simulink model "vehicle5a"  (R2017a)
settings: Solver=VariableStepAuto  StartTime=0.0  StopTime=2  RelTol=1e-3
libraries: elvio x6
settings Model: Creator=tstef  LastModifiedBy=tstef

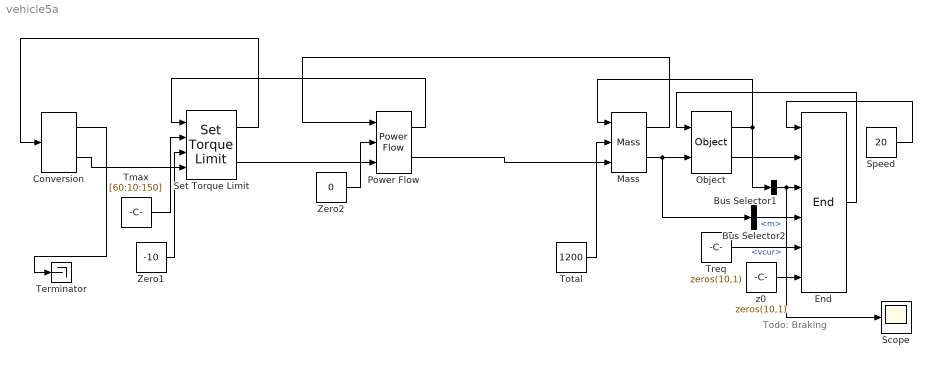
== system vehicle5a ==
  note: Todo: Braking
  Bus Selector1 : BusSelector  OutputSignals=vcur
  Bus Selector2 : BusSelector  OutputSignals=m
  Conversion : elvio/Basics/Conversion
  End : elvio/Basics/End
  Mass : elvio/Basics/Mass
  Object : elvio/Basics/Object
  Power Flow : elvio/Basics/Power Flow
  Scope : Scope
  Set Torque Limit : elvio/Basics/Set Torque Limit
  Speed : Constant  Value=20
  Terminator : Terminator
  Tmax : Constant  Value=[60:10:150]
  Total : Constant  Value=1200
  Treq : Constant  Value=zeros(10,1)
  Zero1 : Constant  Value=-10
  Zero2 : Constant  Value=0
  z0 : Constant  Value=zeros(10,1)
  wires:
  Set Torque Limit/2 -> Power Flow/3
  Conversion/2 -> Set Torque Limit/4
  Speed/1 -> End/1
  Set Torque Limit/1 -> Conversion/1
  Power Flow/1 -> Set Torque Limit/1
  Object/1 -> Mass/1, Bus Selector1/1
  End/1 -> Object/1
  Tmax/1 -> Set Torque Limit/2
  Zero1/1 -> Set Torque Limit/3
  Total/1 -> Mass/2
  Object/2 -> End/2
  Conversion/1 -> Terminator/1
  Bus Selector1/1 -> Scope/1, End/3  "<vcur>"
  Mass/2 -> Bus Selector2/1, Object/2
  z0/1 -> End/6
  Treq/1 -> End/5
  Bus Selector2/1 -> End/4  "<m>"
  Zero2/1 -> Power Flow/2
  Power Flow/2 -> Mass/3
  Mass/1 -> Power Flow/1
